simulink model "Dynamic_RR"  (R2019b)
settings: Solver=VariableStepAuto  StartTime=0.0  StopTime=60  FixedStep=1e-2  RelTol=1e-3
values from neighbouring files (symbols this model uses):
  a = l1+l2*cos_q2    [Inverse_Kinematics.m]    (also in Visual.m = 0.4881; rr_planar_dynamics.m = 0.4)
  A = 0.9972    [Visual.m]    (also in rr_planar_dynamics.m = 0.5)
  B = 1.0044    [Visual.m]    (also in rr_planar_dynamics.m = 1)
  b = l2*sin_q2    [Inverse_Kinematics.m]    (also in Visual.m = 0.223; rr_planar_dynamics.m = 0.8)
  delta = 1.0436    [Visual.m]    (also in rr_planar_dynamics.m = 0.5236)
  fext = zeros(6,3)    [Visual.m]    (also in rr_planar_dynamics.m)
  pi_hat_0 = pi_param*(1+0.01)    [Visual.m]    (also in rr_planar_dynamics.m = pi_param*(1+0.02))
  pi_param = [0.5000; 0.1667; 0.5000; 0.1667]    [Visual.m]    (also in rr_planar_dynamics.m = [1.0000;-0.5000;0.3333;1.0000;-0.5000;0.3333])
libraries: robotmaniplib x1
settings Model: Creator=Stefano  LastModifiedBy=Mardok

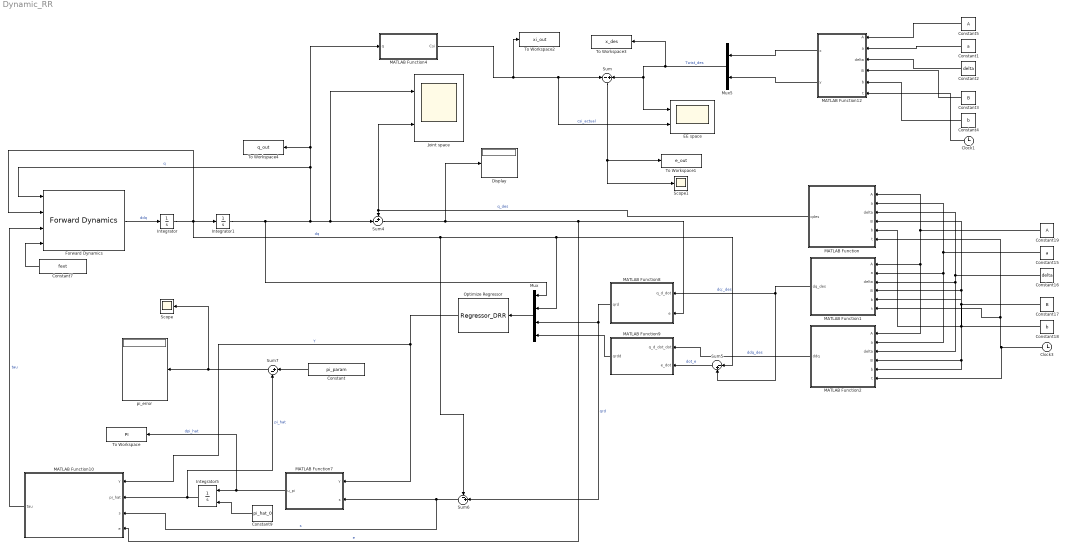
== system Dynamic_RR ==
  Clock1 : Clock
  Clock3 : Clock
  Constant : Constant  Value=pi_param
  Constant1 : Constant  Value=a
  Constant15 : Constant  Value=a
  Constant16 : Constant  Value=delta
  Constant17 : Constant  Value=B
  Constant18 : Constant  Value=b
  Constant19 : Constant  Value=A
  Constant2 : Constant  Value=delta
  Constant3 : Constant  Value=B
  Constant4 : Constant  Value=b
  Constant5 : Constant  Value=A
  Constant7 : Constant  Value=fext
  Constant9 : Constant  Value=pi_hat_0
  Display : Display
  EE space : Scope  NumInputPorts=2
  Forward Dynamics : robotmaniplib/Forward Dynamics  RigidBodyTree=rr  SimulateUsing=Interpreted execution
      settings: SourceProductName=Robotics System Toolbox
  Integrator : Integrator
  Integrator1 : Integrator  InitialCondition=[1.3,4]'
  Integrator5 : Integrator  InitialConditionSource=external
  Joint space : Scope  NumInputPorts=2
  MATLAB Function : MATLAB Function  TreatAsAtomicUnit=on
  MATLAB Function1 : MATLAB Function  TreatAsAtomicUnit=on
  MATLAB Function10 : MATLAB Function  TreatAsAtomicUnit=on
  MATLAB Function12 : MATLAB Function  TreatAsAtomicUnit=on
  MATLAB Function2 : MATLAB Function  TreatAsAtomicUnit=on
  MATLAB Function4 : MATLAB Function  TreatAsAtomicUnit=on
  MATLAB Function7 : MATLAB Function  TreatAsAtomicUnit=on
  MATLAB Function8 : MATLAB Function  TreatAsAtomicUnit=on
  MATLAB Function9 : MATLAB Function  TreatAsAtomicUnit=on
  Mux : Mux
  Mux5 : Mux  Inputs=2
  "Optimize Regressor " : MATLABFcn  MATLABFcn=Regressor_DRR  OutputDimensions=[2,6]  Output1D=off
  Scope : Scope
  Scope1 : Scope
  Sum : Sum  Inputs=-+
  Sum4 : Sum  Inputs=+-|
  Sum5 : Sum  Inputs=|-+
  Sum6 : Sum  Inputs=-+|
  Sum7 : Sum  Inputs=|+-
  To Workspace : ToWorkspace  VariableName=PI  SaveFormat=Timeseries  SampleTime=-1
  To Workspace1 : ToWorkspace  VariableName=e_out  SaveFormat=Timeseries  SampleTime=-1
  To Workspace2 : ToWorkspace  VariableName=xi_out  SaveFormat=Timeseries  SampleTime=-1
  To Workspace3 : ToWorkspace  VariableName=x_des  SaveFormat=Timeseries  SampleTime=-1
  To Workspace4 : ToWorkspace  VariableName=q_out  SaveFormat=Timeseries  SampleTime=-1
  pi_error : Display
  wires:
  Sum6/1 -> MATLAB Function10/3(s), MATLAB Function7/2(s)  "s"
  Sum4/1 -> Display/1, MATLAB Function10/4(e), MATLAB Function8/2(e)  "e"
  Sum5/1 -> MATLAB Function9/2(e_dot)  "dot_e"
  MATLAB Function7/1(u_pi) -> To Workspace/1, Integrator5/1  "dpi_hat"
  Integrator5/1 -> MATLAB Function10/2(pi_hat), Sum7/2  "pi_hat"
  Integrator/1 -> Forward Dynamics/2, Integrator1/1, Mux/2, Sum5/1, Sum6/1  "dq"
  Constant9/1 -> Integrator5/2
  MATLAB Function8/1(qrd) -> Sum6/2, Mux/3  "qrd"
  Mux/1 -> "Optimize Regressor "/1
  MATLAB Function9/1(qrdd) -> Mux/4
  Constant/1 -> Sum7/1
  Sum7/1 -> Scope/1, pi_error/1
  Integrator1/1 -> Mux/1, To Workspace4/1, MATLAB Function4/1(q), Forward Dynamics/1, Joint space/1, Sum4/2  "q"
  MATLAB Function/1(qdes) -> Joint space/2, Sum4/1  "q_des"
  MATLAB Function1/1(dq_des) -> MATLAB Function8/1(q_d_dot), Sum5/2  "dq:_des"
  MATLAB Function2/1(ddq) -> MATLAB Function9/1(q_d_dot_dot)  "ddq_des"
  "Optimize Regressor "/1 -> MATLAB Function10/1(Y), MATLAB Function7/1(Y)  "Y"
  Forward Dynamics/1 -> Integrator/1  "ddq"
  MATLAB Function10/1(tau) -> Forward Dynamics/3  "tau"
  Constant7/1 -> Forward Dynamics/4
  Constant19/1 -> MATLAB Function/1(A), MATLAB Function2/1(A), MATLAB Function1/1(A)
  Constant15/1 -> MATLAB Function/2(a), MATLAB Function2/2(a), MATLAB Function1/2(a)
  Constant16/1 -> MATLAB Function/3(delta), MATLAB Function2/3(delta), MATLAB Function1/3(delta)
  Constant17/1 -> MATLAB Function1/4(B), MATLAB Function/4(B), MATLAB Function2/5(b), MATLAB Function2/4(B)
  Constant18/1 -> MATLAB Function1/5(b), MATLAB Function/5(b)
  Clock3/1 -> MATLAB Function2/6(t), MATLAB Function1/6(t), MATLAB Function/6(t)
  MATLAB Function12/2(y) -> Mux5/2
  MATLAB Function12/1(x) -> Mux5/1
  Constant5/1 -> MATLAB Function12/1(A)
  Constant1/1 -> MATLAB Function12/2(a)
  Constant2/1 -> MATLAB Function12/3(delta)
  Constant3/1 -> MATLAB Function12/4(B)
  Constant4/1 -> MATLAB Function12/5(b)
  Clock1/1 -> MATLAB Function12/6(t)
  MATLAB Function4/1(Csi) -> To Workspace2/1, EE space/2, Sum/1  "csi_actual"
  Mux5/1 -> To Workspace3/1, EE space/1, Sum/2  "Twist_des"
  Sum/1 -> To Workspace1/1, Scope1/1

== matlab function Dynamic_RR/MATLAB Function1 ==
  data: A input; dq_des output; a input; delta input; B input; b input; t input
function dq_des = d_Lissajous(A,a,delta,B,b,t)


dq1 = ((a*cos(delta + a*t)*sin(delta + a*t)*A^2 + b*cos(b*t)*sin(b*t)*B^2)*(1 - ((B^2*sin(b*t)^2)/2 + (A^2*sin(delta + a*t)^2)/2 - 1)^2)^(1/2) + ((a*cos(delta + a*t)*sin(delta + a*t)*A^2 + b*cos(b*t)*sin(b*t)*B^2)*((B^2*sin(b*t)^2)/2 + (A^2*sin(delta + a*t)^2)/2)*((B^2*sin(b*t)^2)/2 + (A^2*sin(delta + a*t)^2)/2 - 1))/(1 - ((A^2*sin(delta + a*t)^2)/2 + (B^2*sin(b*t)^2)/2 - 1)^2)^(1/2))/(((B^2*sin(b*t)^2)/2 + (A^2*sin(delta + a*t)^2)/2)^2 - ((B^2*sin(b*t)^2)/2 + (A^2*sin(delta + a*t)^2)/2 - 1)^2 + 1) - (A*B*a*cos(delta + a*t)*sin(b*t) - A*B*b*sin(delta + a*t)*cos(b*t))/(A^2*sin(delta + a*t)^2 + B^2*sin(b*t)^2);

dq2 = - (a*cos(delta + a*t)*sin(delta + a*t)*A^2 + b*cos(b*t)*sin(b*t)*B^2)*(1 - ((B^2*sin(b*t)^2)/2 + (A^2*sin(delta + a*t)^2)/2 - 1)^2)^(1/2) - ((a*cos(delta + a*t)*sin(delta + a*t)*A^2 + b*cos(b*t)*sin(b*t)*B^2)*((B^2*sin(b*t)^2)/2 + (A^2*sin(delta + a*t)^2)/2 - 1)^2)/(1 - ((A^2*sin(delta + a*t)^2)/2 + (B^2*sin(b*t)^2)/2 - 1)^2)^(1/2);

dq_des = [dq1;dq2];

== matlab function Dynamic_RR/MATLAB Function ==
  data: A input; qdes output; a input; delta input; B input; b input; t input
function qdes = Lissajou(A,a,delta,B,b,t)

q1 = atan2(B*sin(b*t), A*sin(delta + a*t)) - atan2((4 - (A^2*sin(delta + a*t)^2 + B^2*sin(b*t)^2 - 2)^2)^(1/2)/2, (A^2*sin(delta + a*t)^2)/2 + (B^2*sin(b*t)^2)/2);
q2 = atan2((4 - (A^2*sin(delta + a*t)^2 + B^2*sin(b*t)^2 - 2)^2)^(1/2)/2, (A^2*sin(delta + a*t)^2)/2 + (B^2*sin(b*t)^2)/2 - 1);

qdes = [q1;q2];

== matlab function Dynamic_RR/MATLAB Function2 ==
  data: A input; ddq output; a input; delta input; B input; b input; t input
function ddq = dd_Lissajous(A,a,delta,B,b,t)

q1_ddot = (A*B*(a*sin(2*delta + 2*a*t)*A^2 + b*sin(2*b*t)*B^2)*(a*cos(delta + a*t)*sin(b*t) - b*sin(delta + a*t)*cos(b*t)))/(A^2*sin(delta + a*t)^2 + B^2*sin(b*t)^2)^2 - ((a*sin(2*delta + 2*a*t)*A^2 + b*sin(2*b*t)*B^2)*((a*sin(2*delta + 2*a*t)*A^2)/2 + (b*sin(2*b*t)*B^2)/2))/((A^2*sin(delta + a*t)^2 + B^2*sin(b*t)^2)*(4 - (A^2*sin(delta + a*t)^2 + B^2*sin(b*t)^2 - 2)^2)^(1/2)) - (B^6*b^2*(sin(b*t)^4 - 2*sin(b*t)^6) - B^4*b^2*sin(2*b*t)^2 - A^4*a^2*sin(2*delta + 2*a*t)^2 - 4*A^4*a^2*sin(delta + a*t)^2*cos(2*delta + 2*a*t) + A^6*a^2*sin(delta + a*t)^4*cos(2*delta + 2*a*t) + 2*B^4*b^2*cos(2*b*t)*(cos(2*b*t) - 1) - 4*A^2*B^2*a^2*sin(b*t)^2*cos(2*delta + 2*a*t) + A^2*B^4*a^2*sin(b*t)^4*cos(2*delta + 2*a*t) - 4*A^2*B^2*b^2*sin(delta + a*t)^2*cos(2*b*t) + A^4*B^2*b^2*sin(delta + a*t)^4*cos(2*b*t) + 2*A^2*B^4*b^2*sin(delta + a*t)^2*cos(2*b*t)*sin(b*t)^2 - 2*A^2*B^2*a*b*sin(2*b*t)*sin(2*delta + 2*a*t) + 2*A^4*B^2*a^2*sin(delta + a*t)^2*sin(b*t)^2*cos(2*delta + 2*a*t))/(4 - (A^2*sin(delta + a*t)^2 + B^2*sin(b*t)^2 - 2)^2)^(3/2) + (A*B*sin(delta + a*t)*sin(b*t)*(a^2 - b^2))/(A^2*sin(delta + a*t)^2 + B^2*sin(b*t)^2);

q2_ddot = - ((B^2*b^2*cos(2*b*t) + A^2*a^2*cos(2*delta + 2*a*t))*(4 - (A^2*sin(delta + a*t)^2 + B^2*sin(b*t)^2 - 2)^2)^(1/2))/2 - ((a*sin(2*delta + 2*a*t)*A^2 + b*sin(2*b*t)*B^2)^2*((B^2*sin(b*t)^2)/2 + (A^2*sin(delta + a*t)^2)/2 - 1))/(2*(4 - (A^2*sin(delta + a*t)^2 + B^2*sin(b*t)^2 - 2)^2)^(1/2)) - ((a*sin(2*delta + 2*a*t)*A^2 + b*sin(2*b*t)*B^2)^2*(A^2*sin(delta + a*t)^2 + B^2*sin(b*t)^2 - 2)^3)/(4*(4 - (A^2*sin(delta + a*t)^2 + B^2*sin(b*t)^2 - 2)^2)^(3/2)) - ((B^2*b^2*cos(2*b*t) + A^2*a^2*cos(2*delta + 2*a*t))*(A^2*sin(delta + a*t)^2 + B^2*sin(b*t)^2 - 2)^2)/(2*(4 - (A^2*sin(delta + a*t)^2 + B^2*sin(b*t)^2 - 2)^2)^(1/2));

ddq = [q1_ddot; q2_ddot];

== matlab function Dynamic_RR/MATLAB Function12 ==
  data: x output; A input; y output; a input; delta input; B input; b input; t input
function [x,y] = Lissajous(A,a,delta,B,b,t)


x = A*sin(a*t+delta);
y = B*sin(b*t);


end

== matlab function Dynamic_RR/MATLAB Function4 ==
  data: q input; Csi output
function Csi  = Direct_Kinematics_RR(q)

%INPUT: q(1) = q1;
%       q(2) = q2;

%OUTPUT: px = position along x axis
%        py = position along y axis

%Link's lenght

l1 = 1;
l2 = 1;

px = l1 * cos(q(1)) + l2 * cos(q(1)+q(2));
py = l1 * sin(q(1)) + l2 * sin(q(1)+q(2));

Csi = [px; py];
end

== matlab function Dynamic_RR/MATLAB Function10 ==
  data: Y input; tau output; pi_hat input; s input; e input
function tau = Back_Stepping_Control_Law(Y,pi_hat,s,e)

Kd = 10 * eye(2);
Kp = 7 * eye(2);

tau = Y * pi_hat + Kd * s + Kp * e;

end

== matlab function Dynamic_RR/MATLAB Function7 ==
  data: Y input; u_pi output; s input
function u_pi = Update_Law(Y,s)

R = 3*eye(2,6);
u_pi = pinv(R).*(Y.')*s;
end

== matlab function Dynamic_RR/MATLAB Function8 ==
  data: q_d_dot input; qrd output; e input
function qrd = q_r_dot(q_d_dot,e)

lambda = 5  * eye(2);
qrd = q_d_dot + lambda * e;

end

== matlab function Dynamic_RR/MATLAB Function9 ==
  data: q_d_dot_dot input; qrdd output; e_dot input
function qrdd = q_r_dot_dot(q_d_dot_dot,e_dot)

lambda = 5 * eye(2);
qrdd = q_d_dot_dot + lambda*e_dot;

end
